simulink model "CAN_Example"  (R2015b)
settings: Solver=FixedStepDiscrete  StartTime=0.0  StopTime=10.0  RelTol=1e-3
undefined symbols (not defined in the file): CAN429ZGTx_Ex
libraries: CAN_Lib x10, STM32_Config_Lib x1
settings Model: Creator=reynaudp  LastModifiedBy=reynaudp
settings DataIOCC: SaveFormat=Array
settings OptimizationCC: OptimizeModelRefInitCode=on  LifeSpan=1
settings DebuggingCC: SolverPrmCheckMsg=warning
settings HardwareCC: ProdBitPerPointer=32  ProdLargestAtomicInteger=Integer  ProdWordSize=32  ProdHWDeviceType=STMicroelectronics->STM32 32-bit Cortex-M
settings RTWCC: SystemTargetFile=stm32.tlc  TemplateMakefile=stm32.tmf  Description=stm32 (Embedded Target)  GenerateReport=on  Toolchain=Microsoft Windows SDK v7.1 | nmake (64-bit Windows)  IncludeHyperlinkInReport=on
settings CodeAppCC: IgnoreCustomStorageClasses=off  MaxIdLength=64  CustomSymbolStrType=$N$R$M  SimulinkBlockComments=off
settings STFCustomTargetCC: CodeReplacementLibrary=ARM CMSIS SIN COS  ParMdlRefBuildCompliant=on  ConcurrentExecutionCompliant=off  IncludeMdlTerminateFcn=off  GeneratePreprocessorConditionals=Use local settings  CombineOutputUpdateFcns=on  ERTCustomFileBanners=on  SupportContinuousTime=off  SupportNonInlinedSFcns=off  MATLABClassNameForMDSCustomization=Simulink.SoftwareTarget.ERTCustomization  CPPClassGenCompliant=off  GRTInterface=off  SystemTargetFile=stm32.tlc
settings ERTTargetCC: CodeReplacementLibrary=ARM CMSIS SIN COS  CompOptLevelCompliant=off  ConcurrentExecutionCompliant=off  IncludeMdlTerminateFcn=off  ERTFirstTimeCompliant=off  ModelStepFunctionPrototypeControlCompliant=off  CPPClassGenCompliant=off  UseToolchainInfoCompliant=off  ERTSrcFileBannerTemplate=sourceFileTemplate.cgt  ERTHdrFileBannerTemplate=sourceFileTemplate.cgt  ERTDataSrcFileTemplate=sourceFileTemplate.cgt  ERTDataHdrFileTemplate=sourceFileTemplate.cgt  ERTCustomFileTemplate=customRoutineProcess.tlc
settings ConfigComp: CovModelRefEnable=Off  CovSFcnEnable=off

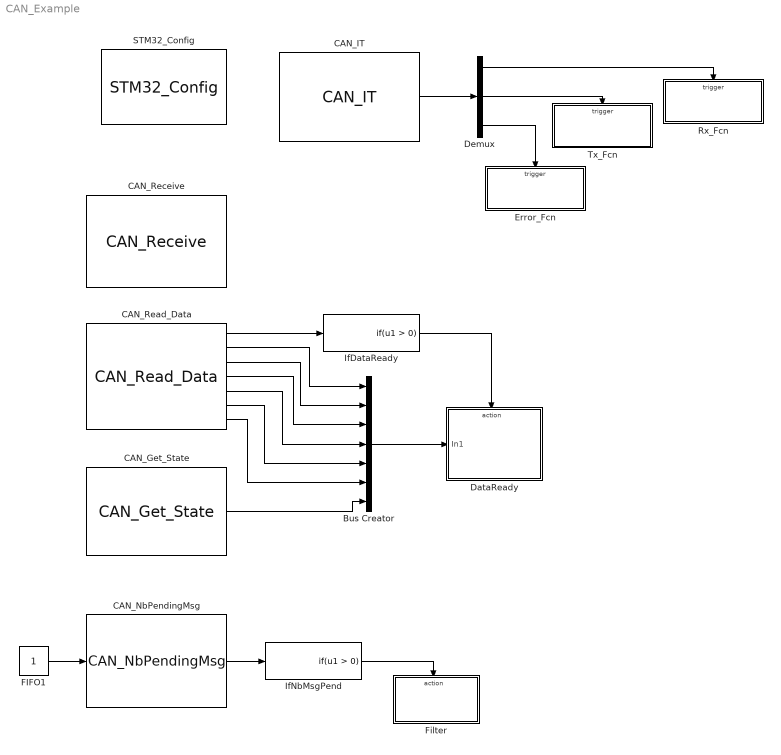
== system CAN_Example ==
  Bus Creator : BusCreator  Inputs=7
  CAN_Get_State : CAN_Lib/CAN_Get_State  CAN_name=CAN1  nbCAN=0
  CAN_IT : CAN_Lib/CAN_IT  CAN_name=CAN1  CAN_Mode=Master  CAN_It=on  CAN_RX_It=on  CAN_TX_It=on  CAN_ERROR_It=on  nbCAN=2
  CAN_NbPendingMsg : CAN_Lib/CAN_NbPendingMsg  CAN_name=CAN1  CAN_Fifo=CAN_FIFO0  CAN_FifoNum=on  CAN_It=on  CAN_Mode=Master  nbCAN=2
  CAN_Read_Data : CAN_Lib/CAN_Read_Data  CAN_name=CAN1  nbCAN=0
  CAN_Receive : CAN_Lib/CAN_Receive  CAN_name=CAN1  CAN_Fifo=CAN_FIFO1  CAN_It=on  CAN_Rcv_TimeOut=10  CAN_Mode=Master  nbCAN=2  CAN_TXT=Interrupt mode. Data available from CAN_Read_Data block model.
  DataReady : Subsystem  TreatAsAtomicUnit=on
  Demux : Demux  Outputs=3
  Error_Fcn : Subsystem  TreatAsAtomicUnit=on
  FIFO1 : Constant
  Filter : Subsystem  TreatAsAtomicUnit=on
  IfDataReady : If  ShowElse=off
  IfNbMsgPend : If  ShowElse=off
  Rx_Fcn : Subsystem  TreatAsAtomicUnit=on
  STM32_Config : STM32_Config_Lib/STM32_Config  Priority=0  Project_Path=.\CAN429ZGTx_Ex\  Config_File=CAN429ZGTx_Ex.ioc  MCU_Name=STM32F429ZGTx
  Tx_Fcn : Subsystem  TreatAsAtomicUnit=on
  wires:
  CAN_IT/1 -> Demux/1
  Demux/1 -> Rx_Fcn/Trigger
  Demux/2 -> Tx_Fcn/Trigger
  Demux/3 -> Error_Fcn/Trigger
  IfDataReady/1 -> DataReady/Action
  CAN_Read_Data/2 -> Bus Creator/1
  CAN_Read_Data/3 -> Bus Creator/2
  CAN_Read_Data/4 -> Bus Creator/3
  CAN_Read_Data/5 -> Bus Creator/4
  CAN_Read_Data/6 -> Bus Creator/5
  CAN_Read_Data/7 -> Bus Creator/6
  Bus Creator/1 -> DataReady/1(In1)
  CAN_Get_State/1 -> Bus Creator/7
  FIFO1/1 -> CAN_NbPendingMsg/1
  CAN_NbPendingMsg/1 -> IfNbMsgPend/1
  IfNbMsgPend/1 -> Filter/Action
  CAN_Read_Data/1 -> IfDataReady/1

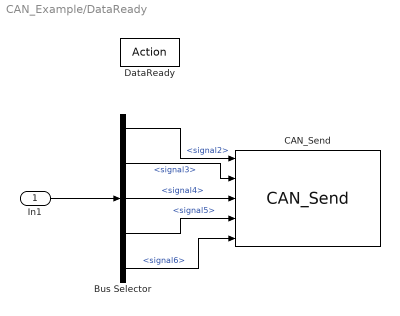
== system CAN_Example/DataReady ==
  In1 : Inport
  DataReady : ActionPort  ActionType=then
  Bus Selector : BusSelector  OutputSignals=signal2,signal3,signal4,signal5,signal6
  CAN_Send : CAN_Lib/CAN_Send  CAN_name=CAN1  CAN_It=on  CAN_Send_TimeOut=10  CAN_Mode=Master  nbCAN=2
  wires:
  In1/1 -> Bus Selector/1
  Bus Selector/1 -> CAN_Send/1  "<signal2>"
  Bus Selector/2 -> CAN_Send/2  "<signal3>"
  Bus Selector/3 -> CAN_Send/3  "<signal4>"
  Bus Selector/4 -> CAN_Send/4  "<signal5>"
  Bus Selector/5 -> CAN_Send/5  "<signal6>"

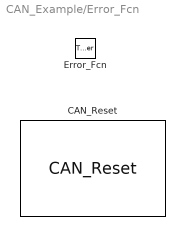
== system CAN_Example/Error_Fcn ==
  Error_Fcn : TriggerPort  TriggerType=function-call
  CAN_Reset : CAN_Lib/CAN_Reset  CAN_name=CAN1  CAN_It=on  CAN_Mode=Master  nbCAN=2

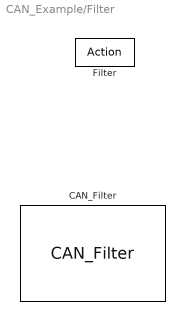
== system CAN_Example/Filter ==
  Filter : ActionPort  ActionType=then
  CAN_Filter : CAN_Lib/CAN_Filter  CAN_name=CAN1  CAN_Enable=on  CAN_Fifo=CAN_FIFO1  CAN_Id_High=12  CAN_Id_Low=14  CAN_Mask_Id_High=1  CAN_Mask_Id_Low=2  CAN_Filter_Number=5  CAN_Mode=CAN_FILTERMODE_IDLIST  CAN_Filter_Scale=CAN_FILTERSCALE_32BIT  CAN_Bank_Number=4  nbCAN=0

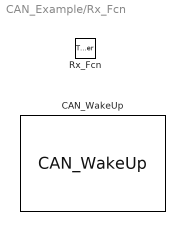
== system CAN_Example/Rx_Fcn ==
  Rx_Fcn : TriggerPort  TriggerType=function-call
  CAN_WakeUp : CAN_Lib/CAN_WakeUp  CAN_name=CAN1  CAN_It=on  CAN_Mode=Master  nbCAN=2

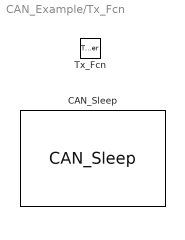
== system CAN_Example/Tx_Fcn ==
  Tx_Fcn : TriggerPort  TriggerType=function-call
  CAN_Sleep : CAN_Lib/CAN_Sleep  CAN_name=CAN1  CAN_It=on  CAN_Mode=Master  nbCAN=2
